simulink model "gm_FCS_MPC_3Phase_SPMSM_TEST1"  (R2022a)
settings: Solver=ode23t  StartTime=0.0  StopTime=0.2  RelTol=1e-3  AbsTol=1e-3  EnableMultiTasking=on
undefined symbols (not defined in the file or in its folder): f_c, Ld, Lq, np, psiPM, R, T_50MHz, u_dc
libraries: hdlmdlgenlib x26, ee_lib x22, nesl_utility x22, fl_lib x21, simulink x7
(part 4 of 5)

== system gm_FCS_MPC_3Phase_SPMSM_TEST1/Microcontroller Software/Subsystem1/MATLAB Function/adder25 ==
  In1 : Inport
  In2 : Inport  Port=2
  adder25 : Sum  OutDataTypeStr=single  SampleTime=1e-08
  Out1 : Outport
  wires:
  In1/1 -> adder25/1
  In2/1 -> adder25/2
  adder25/1 -> Out1/1

== system gm_FCS_MPC_3Phase_SPMSM_TEST1/Microcontroller Software/Subsystem1/MATLAB Function/adder26 ==
  In1 : Inport
  In2 : Inport  Port=2
  adder26 : Sum  OutDataTypeStr=single  SampleTime=1e-08
  Out1 : Outport
  wires:
  In1/1 -> adder26/1
  In2/1 -> adder26/2
  adder26/1 -> Out1/1

== system gm_FCS_MPC_3Phase_SPMSM_TEST1/Microcontroller Software/Subsystem1/MATLAB Function/adder27 ==
  In1 : Inport
  In2 : Inport  Port=2
  adder27 : Sum  OutDataTypeStr=single  SampleTime=1e-08
  Out1 : Outport
  wires:
  In1/1 -> adder27/1
  In2/1 -> adder27/2
  adder27/1 -> Out1/1

== system gm_FCS_MPC_3Phase_SPMSM_TEST1/Microcontroller Software/Subsystem1/MATLAB Function/adder28 ==
  In1 : Inport
  In2 : Inport  Port=2
  adder28 : Sum  OutDataTypeStr=single  SampleTime=1e-08
  Out1 : Outport
  wires:
  In1/1 -> adder28/1
  In2/1 -> adder28/2
  adder28/1 -> Out1/1

== system gm_FCS_MPC_3Phase_SPMSM_TEST1/Microcontroller Software/Subsystem1/MATLAB Function/adder29 ==
  In1 : Inport
  In2 : Inport  Port=2
  adder29 : Sum  OutDataTypeStr=single  SampleTime=1e-08
  Out1 : Outport
  wires:
  In1/1 -> adder29/1
  In2/1 -> adder29/2
  adder29/1 -> Out1/1

== system gm_FCS_MPC_3Phase_SPMSM_TEST1/Microcontroller Software/Subsystem1/MATLAB Function/adder3 ==
  In1 : Inport
  In2 : Inport  Port=2
  adder3 : Sum  OutDataTypeStr=single  SampleTime=1e-08
  Out1 : Outport
  wires:
  In1/1 -> adder3/1
  In2/1 -> adder3/2
  adder3/1 -> Out1/1

== system gm_FCS_MPC_3Phase_SPMSM_TEST1/Microcontroller Software/Subsystem1/MATLAB Function/adder30 ==
  In1 : Inport
  In2 : Inport  Port=2
  adder30 : Sum  OutDataTypeStr=single  SampleTime=1e-08
  Out1 : Outport
  wires:
  In1/1 -> adder30/1
  In2/1 -> adder30/2
  adder30/1 -> Out1/1

== system gm_FCS_MPC_3Phase_SPMSM_TEST1/Microcontroller Software/Subsystem1/MATLAB Function/adder31 ==
  In1 : Inport
  In2 : Inport  Port=2
  adder31 : Sum  OutDataTypeStr=single  SampleTime=1e-08
  Out1 : Outport
  wires:
  In1/1 -> adder31/1
  In2/1 -> adder31/2
  adder31/1 -> Out1/1

== system gm_FCS_MPC_3Phase_SPMSM_TEST1/Microcontroller Software/Subsystem1/MATLAB Function/adder32 ==
  In1 : Inport
  In2 : Inport  Port=2
  adder32 : Sum  OutDataTypeStr=single  SampleTime=1e-08
  Out1 : Outport
  wires:
  In1/1 -> adder32/1
  In2/1 -> adder32/2
  adder32/1 -> Out1/1

== system gm_FCS_MPC_3Phase_SPMSM_TEST1/Microcontroller Software/Subsystem1/MATLAB Function/adder33 ==
  In1 : Inport
  In2 : Inport  Port=2
  adder33 : Sum  OutDataTypeStr=single  SampleTime=1e-08
  Out1 : Outport
  wires:
  In1/1 -> adder33/1
  In2/1 -> adder33/2
  adder33/1 -> Out1/1

== system gm_FCS_MPC_3Phase_SPMSM_TEST1/Microcontroller Software/Subsystem1/MATLAB Function/adder34 ==
  In1 : Inport
  In2 : Inport  Port=2
  adder34 : Sum  OutDataTypeStr=single  SampleTime=1e-08
  Out1 : Outport
  wires:
  In1/1 -> adder34/1
  In2/1 -> adder34/2
  adder34/1 -> Out1/1

== system gm_FCS_MPC_3Phase_SPMSM_TEST1/Microcontroller Software/Subsystem1/MATLAB Function/adder4 ==
  In1 : Inport
  In2 : Inport  Port=2
  adder4 : Sum  OutDataTypeStr=single  SampleTime=1e-08
  Out1 : Outport
  wires:
  In1/1 -> adder4/1
  In2/1 -> adder4/2
  adder4/1 -> Out1/1

== system gm_FCS_MPC_3Phase_SPMSM_TEST1/Microcontroller Software/Subsystem1/MATLAB Function/adder5 ==
  In1 : Inport
  In2 : Inport  Port=2
  adder5 : Sum  OutDataTypeStr=single  SampleTime=1e-08
  Out1 : Outport
  wires:
  In1/1 -> adder5/1
  In2/1 -> adder5/2
  adder5/1 -> Out1/1

== system gm_FCS_MPC_3Phase_SPMSM_TEST1/Microcontroller Software/Subsystem1/MATLAB Function/adder6 ==
  In1 : Inport
  In2 : Inport  Port=2
  adder6 : Sum  OutDataTypeStr=single  SampleTime=1e-08
  Out1 : Outport
  wires:
  In1/1 -> adder6/1
  In2/1 -> adder6/2
  adder6/1 -> Out1/1

== system gm_FCS_MPC_3Phase_SPMSM_TEST1/Microcontroller Software/Subsystem1/MATLAB Function/adder7 ==
  In1 : Inport
  In2 : Inport  Port=2
  adder7 : Sum  OutDataTypeStr=single  SampleTime=1e-08
  Out1 : Outport
  wires:
  In1/1 -> adder7/1
  In2/1 -> adder7/2
  adder7/1 -> Out1/1

== system gm_FCS_MPC_3Phase_SPMSM_TEST1/Microcontroller Software/Subsystem1/MATLAB Function/adder8 ==
  In1 : Inport
  In2 : Inport  Port=2
  adder8 : Sum  OutDataTypeStr=single  SampleTime=1e-08
  Out1 : Outport
  wires:
  In1/1 -> adder8/1
  In2/1 -> adder8/2
  adder8/1 -> Out1/1

== system gm_FCS_MPC_3Phase_SPMSM_TEST1/Microcontroller Software/Subsystem1/MATLAB Function/adder9 ==
  In1 : Inport
  In2 : Inport  Port=2
  adder9 : Sum  OutDataTypeStr=single  SampleTime=1e-08
  Out1 : Outport
  wires:
  In1/1 -> adder9/1
  In2/1 -> adder9/2
  adder9/1 -> Out1/1

== system gm_FCS_MPC_3Phase_SPMSM_TEST1/Microcontroller Software/Subsystem1/MATLAB Function/cos_to_sincos ==
  In1 : Inport
  cos_to_sincos : Trigonometry  Operator=sincos  SampleTime=1e-08
  Out1 : Outport
  Out2 : Outport  Port=2
  wires:
  In1/1 -> cos_to_sincos/1
  cos_to_sincos/1 -> Out1/1
  cos_to_sincos/2 -> Out2/1

== system gm_FCS_MPC_3Phase_SPMSM_TEST1/Microcontroller Software/Subsystem1/MATLAB Function/divider ==
  In1 : Inport
  In2 : Inport  Port=2
  divider : Product  Inputs=*/  OutDataTypeStr=single  SampleTime=1e-08
  Out1 : Outport
  wires:
  In1/1 -> divider/1
  In2/1 -> divider/2
  divider/1 -> Out1/1

== system gm_FCS_MPC_3Phase_SPMSM_TEST1/Microcontroller Software/Subsystem1/MATLAB Function/divider1 ==
  In1 : Inport
  In2 : Inport  Port=2
  divider1 : Product  Inputs=*/  OutDataTypeStr=single  SampleTime=1e-08
  Out1 : Outport
  wires:
  In1/1 -> divider1/1
  In2/1 -> divider1/2
  divider1/1 -> Out1/1

== system gm_FCS_MPC_3Phase_SPMSM_TEST1/Microcontroller Software/Subsystem1/MATLAB Function/divider10 ==
  In1 : Inport
  In2 : Inport  Port=2
  divider10 : Product  Inputs=*/  OutDataTypeStr=single  SampleTime=1e-08
  Out1 : Outport
  wires:
  In1/1 -> divider10/1
  In2/1 -> divider10/2
  divider10/1 -> Out1/1

== system gm_FCS_MPC_3Phase_SPMSM_TEST1/Microcontroller Software/Subsystem1/MATLAB Function/divider11 ==
  In1 : Inport
  In2 : Inport  Port=2
  divider11 : Product  Inputs=*/  OutDataTypeStr=single  SampleTime=1e-08
  Out1 : Outport
  wires:
  In1/1 -> divider11/1
  In2/1 -> divider11/2
  divider11/1 -> Out1/1

== system gm_FCS_MPC_3Phase_SPMSM_TEST1/Microcontroller Software/Subsystem1/MATLAB Function/divider12 ==
  In1 : Inport
  In2 : Inport  Port=2
  divider12 : Product  Inputs=*/  OutDataTypeStr=single  SampleTime=1e-08
  Out1 : Outport
  wires:
  In1/1 -> divider12/1
  In2/1 -> divider12/2
  divider12/1 -> Out1/1

== system gm_FCS_MPC_3Phase_SPMSM_TEST1/Microcontroller Software/Subsystem1/MATLAB Function/divider13 ==
  In1 : Inport
  In2 : Inport  Port=2
  divider13 : Product  Inputs=*/  OutDataTypeStr=single  SampleTime=1e-08
  Out1 : Outport
  wires:
  In1/1 -> divider13/1
  In2/1 -> divider13/2
  divider13/1 -> Out1/1

== system gm_FCS_MPC_3Phase_SPMSM_TEST1/Microcontroller Software/Subsystem1/MATLAB Function/divider14 ==
  In1 : Inport
  In2 : Inport  Port=2
  divider14 : Product  Inputs=*/  OutDataTypeStr=single  SampleTime=1e-08
  Out1 : Outport
  wires:
  In1/1 -> divider14/1
  In2/1 -> divider14/2
  divider14/1 -> Out1/1

== system gm_FCS_MPC_3Phase_SPMSM_TEST1/Microcontroller Software/Subsystem1/MATLAB Function/divider15 ==
  In1 : Inport
  In2 : Inport  Port=2
  divider15 : Product  Inputs=*/  OutDataTypeStr=single  SampleTime=1e-08
  Out1 : Outport
  wires:
  In1/1 -> divider15/1
  In2/1 -> divider15/2
  divider15/1 -> Out1/1

== system gm_FCS_MPC_3Phase_SPMSM_TEST1/Microcontroller Software/Subsystem1/MATLAB Function/divider16 ==
  In1 : Inport
  In2 : Inport  Port=2
  divider16 : Product  Inputs=*/  OutDataTypeStr=single  SampleTime=1e-08
  Out1 : Outport
  wires:
  In1/1 -> divider16/1
  In2/1 -> divider16/2
  divider16/1 -> Out1/1

== system gm_FCS_MPC_3Phase_SPMSM_TEST1/Microcontroller Software/Subsystem1/MATLAB Function/divider17 ==
  In1 : Inport
  In2 : Inport  Port=2
  divider17 : Product  Inputs=*/  OutDataTypeStr=single  SampleTime=1e-08
  Out1 : Outport
  wires:
  In1/1 -> divider17/1
  In2/1 -> divider17/2
  divider17/1 -> Out1/1

== system gm_FCS_MPC_3Phase_SPMSM_TEST1/Microcontroller Software/Subsystem1/MATLAB Function/divider18 ==
  In1 : Inport
  In2 : Inport  Port=2
  divider18 : Product  Inputs=*/  OutDataTypeStr=single  SampleTime=1e-08
  Out1 : Outport
  wires:
  In1/1 -> divider18/1
  In2/1 -> divider18/2
  divider18/1 -> Out1/1

== system gm_FCS_MPC_3Phase_SPMSM_TEST1/Microcontroller Software/Subsystem1/MATLAB Function/divider19 ==
  In1 : Inport
  In2 : Inport  Port=2
  divider19 : Product  Inputs=*/  OutDataTypeStr=single  SampleTime=1e-08
  Out1 : Outport
  wires:
  In1/1 -> divider19/1
  In2/1 -> divider19/2
  divider19/1 -> Out1/1

== system gm_FCS_MPC_3Phase_SPMSM_TEST1/Microcontroller Software/Subsystem1/MATLAB Function/divider2 ==
  In1 : Inport
  In2 : Inport  Port=2
  divider2 : Product  Inputs=*/  OutDataTypeStr=single  SampleTime=1e-08
  Out1 : Outport
  wires:
  In1/1 -> divider2/1
  In2/1 -> divider2/2
  divider2/1 -> Out1/1

== system gm_FCS_MPC_3Phase_SPMSM_TEST1/Microcontroller Software/Subsystem1/MATLAB Function/divider20 ==
  In1 : Inport
  In2 : Inport  Port=2
  divider20 : Product  Inputs=*/  OutDataTypeStr=single  SampleTime=1e-08
  Out1 : Outport
  wires:
  In1/1 -> divider20/1
  In2/1 -> divider20/2
  divider20/1 -> Out1/1

== system gm_FCS_MPC_3Phase_SPMSM_TEST1/Microcontroller Software/Subsystem1/MATLAB Function/divider21 ==
  In1 : Inport
  In2 : Inport  Port=2
  divider21 : Product  Inputs=*/  OutDataTypeStr=single  SampleTime=1e-08
  Out1 : Outport
  wires:
  In1/1 -> divider21/1
  In2/1 -> divider21/2
  divider21/1 -> Out1/1

== system gm_FCS_MPC_3Phase_SPMSM_TEST1/Microcontroller Software/Subsystem1/MATLAB Function/divider22 ==
  In1 : Inport
  In2 : Inport  Port=2
  divider22 : Product  Inputs=*/  OutDataTypeStr=single  SampleTime=1e-08
  Out1 : Outport
  wires:
  In1/1 -> divider22/1
  In2/1 -> divider22/2
  divider22/1 -> Out1/1

== system gm_FCS_MPC_3Phase_SPMSM_TEST1/Microcontroller Software/Subsystem1/MATLAB Function/divider23 ==
  In1 : Inport
  In2 : Inport  Port=2
  divider23 : Product  Inputs=*/  OutDataTypeStr=single  SampleTime=1e-08
  Out1 : Outport
  wires:
  In1/1 -> divider23/1
  In2/1 -> divider23/2
  divider23/1 -> Out1/1

== system gm_FCS_MPC_3Phase_SPMSM_TEST1/Microcontroller Software/Subsystem1/MATLAB Function/divider24 ==
  In1 : Inport
  In2 : Inport  Port=2
  divider24 : Product  Inputs=*/  OutDataTypeStr=single  SampleTime=1e-08
  Out1 : Outport
  wires:
  In1/1 -> divider24/1
  In2/1 -> divider24/2
  divider24/1 -> Out1/1

== system gm_FCS_MPC_3Phase_SPMSM_TEST1/Microcontroller Software/Subsystem1/MATLAB Function/divider25 ==
  In1 : Inport
  In2 : Inport  Port=2
  divider25 : Product  Inputs=*/  OutDataTypeStr=single  SampleTime=1e-08
  Out1 : Outport
  wires:
  In1/1 -> divider25/1
  In2/1 -> divider25/2
  divider25/1 -> Out1/1

== system gm_FCS_MPC_3Phase_SPMSM_TEST1/Microcontroller Software/Subsystem1/MATLAB Function/divider26 ==
  In1 : Inport
  In2 : Inport  Port=2
  divider26 : Product  Inputs=*/  OutDataTypeStr=single  SampleTime=1e-08
  Out1 : Outport
  wires:
  In1/1 -> divider26/1
  In2/1 -> divider26/2
  divider26/1 -> Out1/1

== system gm_FCS_MPC_3Phase_SPMSM_TEST1/Microcontroller Software/Subsystem1/MATLAB Function/divider27 ==
  In1 : Inport
  In2 : Inport  Port=2
  divider27 : Product  Inputs=*/  OutDataTypeStr=single  SampleTime=1e-08
  Out1 : Outport
  wires:
  In1/1 -> divider27/1
  In2/1 -> divider27/2
  divider27/1 -> Out1/1

== system gm_FCS_MPC_3Phase_SPMSM_TEST1/Microcontroller Software/Subsystem1/MATLAB Function/divider28 ==
  In1 : Inport
  In2 : Inport  Port=2
  divider28 : Product  Inputs=*/  OutDataTypeStr=single  SampleTime=1e-08
  Out1 : Outport
  wires:
  In1/1 -> divider28/1
  In2/1 -> divider28/2
  divider28/1 -> Out1/1

== system gm_FCS_MPC_3Phase_SPMSM_TEST1/Microcontroller Software/Subsystem1/MATLAB Function/divider29 ==
  In1 : Inport
  In2 : Inport  Port=2
  divider29 : Product  Inputs=*/  OutDataTypeStr=single  SampleTime=1e-08
  Out1 : Outport
  wires:
  In1/1 -> divider29/1
  In2/1 -> divider29/2
  divider29/1 -> Out1/1

== system gm_FCS_MPC_3Phase_SPMSM_TEST1/Microcontroller Software/Subsystem1/MATLAB Function/divider3 ==
  In1 : Inport
  In2 : Inport  Port=2
  divider3 : Product  Inputs=*/  OutDataTypeStr=single  SampleTime=1e-08
  Out1 : Outport
  wires:
  In1/1 -> divider3/1
  In2/1 -> divider3/2
  divider3/1 -> Out1/1

== system gm_FCS_MPC_3Phase_SPMSM_TEST1/Microcontroller Software/Subsystem1/MATLAB Function/divider30 ==
  In1 : Inport
  In2 : Inport  Port=2
  divider30 : Product  Inputs=*/  OutDataTypeStr=single  SampleTime=1e-08
  Out1 : Outport
  wires:
  In1/1 -> divider30/1
  In2/1 -> divider30/2
  divider30/1 -> Out1/1

== system gm_FCS_MPC_3Phase_SPMSM_TEST1/Microcontroller Software/Subsystem1/MATLAB Function/divider31 ==
  In1 : Inport
  In2 : Inport  Port=2
  divider31 : Product  Inputs=*/  OutDataTypeStr=single  SampleTime=1e-08
  Out1 : Outport
  wires:
  In1/1 -> divider31/1
  In2/1 -> divider31/2
  divider31/1 -> Out1/1

== system gm_FCS_MPC_3Phase_SPMSM_TEST1/Microcontroller Software/Subsystem1/MATLAB Function/divider32 ==
  In1 : Inport
  In2 : Inport  Port=2
  divider32 : Product  Inputs=*/  OutDataTypeStr=single  SampleTime=1e-08
  Out1 : Outport
  wires:
  In1/1 -> divider32/1
  In2/1 -> divider32/2
  divider32/1 -> Out1/1

== system gm_FCS_MPC_3Phase_SPMSM_TEST1/Microcontroller Software/Subsystem1/MATLAB Function/divider33 ==
  In1 : Inport
  In2 : Inport  Port=2
  divider33 : Product  Inputs=*/  OutDataTypeStr=single  SampleTime=1e-08
  Out1 : Outport
  wires:
  In1/1 -> divider33/1
  In2/1 -> divider33/2
  divider33/1 -> Out1/1

== system gm_FCS_MPC_3Phase_SPMSM_TEST1/Microcontroller Software/Subsystem1/MATLAB Function/divider34 ==
  In1 : Inport
  In2 : Inport  Port=2
  divider34 : Product  Inputs=*/  OutDataTypeStr=single  SampleTime=1e-08
  Out1 : Outport
  wires:
  In1/1 -> divider34/1
  In2/1 -> divider34/2
  divider34/1 -> Out1/1

== system gm_FCS_MPC_3Phase_SPMSM_TEST1/Microcontroller Software/Subsystem1/MATLAB Function/divider35 ==
  In1 : Inport
  In2 : Inport  Port=2
  divider35 : Product  Inputs=*/  OutDataTypeStr=single  SampleTime=1e-08
  Out1 : Outport
  wires:
  In1/1 -> divider35/1
  In2/1 -> divider35/2
  divider35/1 -> Out1/1

== system gm_FCS_MPC_3Phase_SPMSM_TEST1/Microcontroller Software/Subsystem1/MATLAB Function/divider4 ==
  In1 : Inport
  In2 : Inport  Port=2
  divider4 : Product  Inputs=*/  OutDataTypeStr=single  SampleTime=1e-08
  Out1 : Outport
  wires:
  In1/1 -> divider4/1
  In2/1 -> divider4/2
  divider4/1 -> Out1/1

== system gm_FCS_MPC_3Phase_SPMSM_TEST1/Microcontroller Software/Subsystem1/MATLAB Function/divider5 ==
  In1 : Inport
  In2 : Inport  Port=2
  divider5 : Product  Inputs=*/  OutDataTypeStr=single  SampleTime=1e-08
  Out1 : Outport
  wires:
  In1/1 -> divider5/1
  In2/1 -> divider5/2
  divider5/1 -> Out1/1

== system gm_FCS_MPC_3Phase_SPMSM_TEST1/Microcontroller Software/Subsystem1/MATLAB Function/divider6 ==
  In1 : Inport
  In2 : Inport  Port=2
  divider6 : Product  Inputs=*/  OutDataTypeStr=single  SampleTime=1e-08
  Out1 : Outport
  wires:
  In1/1 -> divider6/1
  In2/1 -> divider6/2
  divider6/1 -> Out1/1

== system gm_FCS_MPC_3Phase_SPMSM_TEST1/Microcontroller Software/Subsystem1/MATLAB Function/divider7 ==
  In1 : Inport
  In2 : Inport  Port=2
  divider7 : Product  Inputs=*/  OutDataTypeStr=single  SampleTime=1e-08
  Out1 : Outport
  wires:
  In1/1 -> divider7/1
  In2/1 -> divider7/2
  divider7/1 -> Out1/1

== system gm_FCS_MPC_3Phase_SPMSM_TEST1/Microcontroller Software/Subsystem1/MATLAB Function/divider8 ==
  In1 : Inport
  In2 : Inport  Port=2
  divider8 : Product  Inputs=*/  OutDataTypeStr=single  SampleTime=1e-08
  Out1 : Outport
  wires:
  In1/1 -> divider8/1
  In2/1 -> divider8/2
  divider8/1 -> Out1/1

== system gm_FCS_MPC_3Phase_SPMSM_TEST1/Microcontroller Software/Subsystem1/MATLAB Function/divider9 ==
  In1 : Inport
  In2 : Inport  Port=2
  divider9 : Product  Inputs=*/  OutDataTypeStr=single  SampleTime=1e-08
  Out1 : Outport
  wires:
  In1/1 -> divider9/1
  In2/1 -> divider9/2
  divider9/1 -> Out1/1

== system gm_FCS_MPC_3Phase_SPMSM_TEST1/Microcontroller Software/Subsystem1/MATLAB Function/dtc ==
  In1 : Inport
  dtc : DataTypeConversion  OutDataTypeStr=double  SampleTime=1e-08  SaturateOnIntegerOverflow=off  RndMeth=Floor
  Out1 : Outport
  wires:
  In1/1 -> dtc/1
  dtc/1 -> Out1/1

== system gm_FCS_MPC_3Phase_SPMSM_TEST1/Microcontroller Software/Subsystem1/MATLAB Function/dtc1 ==
  In1 : Inport
  dtc1 : DataTypeConversion  OutDataTypeStr=double  SampleTime=1e-08  SaturateOnIntegerOverflow=off  RndMeth=Floor
  Out1 : Outport
  wires:
  In1/1 -> dtc1/1
  dtc1/1 -> Out1/1

== system gm_FCS_MPC_3Phase_SPMSM_TEST1/Microcontroller Software/Subsystem1/MATLAB Function/dtc2 ==
  In1 : Inport
  dtc2 : DataTypeConversion  OutDataTypeStr=double  SampleTime=1e-08  SaturateOnIntegerOverflow=off  RndMeth=Floor
  Out1 : Outport
  wires:
  In1/1 -> dtc2/1
  dtc2/1 -> Out1/1

== system gm_FCS_MPC_3Phase_SPMSM_TEST1/Microcontroller Software/Subsystem1/MATLAB Function/dtc3 ==
  In1 : Inport
  dtc3 : DataTypeConversion  OutDataTypeStr=double  SampleTime=1e-08  SaturateOnIntegerOverflow=off  RndMeth=Floor
  Out1 : Outport
  wires:
  In1/1 -> dtc3/1
  dtc3/1 -> Out1/1

== system gm_FCS_MPC_3Phase_SPMSM_TEST1/Microcontroller Software/Subsystem1/MATLAB Function/dtc4 ==
  In1 : Inport
  dtc4 : DataTypeConversion  OutDataTypeStr=double  SampleTime=1e-08  SaturateOnIntegerOverflow=off  RndMeth=Floor
  Out1 : Outport
  wires:
  In1/1 -> dtc4/1
  dtc4/1 -> Out1/1

== system gm_FCS_MPC_3Phase_SPMSM_TEST1/Microcontroller Software/Subsystem1/MATLAB Function/dtc5 ==
  In1 : Inport
  dtc5 : DataTypeConversion  OutDataTypeStr=double  SampleTime=1e-08  SaturateOnIntegerOverflow=off  RndMeth=Floor
  Out1 : Outport
  wires:
  In1/1 -> dtc5/1
  dtc5/1 -> Out1/1

== system gm_FCS_MPC_3Phase_SPMSM_TEST1/Microcontroller Software/Subsystem1/MATLAB Function/dtc6 ==
  In1 : Inport
  dtc6 : DataTypeConversion  OutDataTypeStr=double  SampleTime=1e-08  SaturateOnIntegerOverflow=off  RndMeth=Floor
  Out1 : Outport
  wires:
  In1/1 -> dtc6/1
  dtc6/1 -> Out1/1

== system gm_FCS_MPC_3Phase_SPMSM_TEST1/Microcontroller Software/Subsystem1/MATLAB Function/dtc7 ==
  In1 : Inport
  dtc7 : DataTypeConversion  OutDataTypeStr=double  SampleTime=1e-08  SaturateOnIntegerOverflow=off  RndMeth=Floor
  Out1 : Outport
  wires:
  In1/1 -> dtc7/1
  dtc7/1 -> Out1/1

== system gm_FCS_MPC_3Phase_SPMSM_TEST1/Microcontroller Software/Subsystem1/MATLAB Function/gain1 ==
  In1 : Inport
  In2 : Inport  Port=2
  gain1 : Product  Inputs=**  OutDataTypeStr=single  SampleTime=1e-08
  Out1 : Outport
  wires:
  In1/1 -> gain1/1
  In2/1 -> gain1/2
  gain1/1 -> Out1/1

== system gm_FCS_MPC_3Phase_SPMSM_TEST1/Microcontroller Software/Subsystem1/MATLAB Function/multiplier ==
  In1 : Inport
  In2 : Inport  Port=2
  multiplier : Product  Inputs=**  OutDataTypeStr=single  SampleTime=1e-08
  Out1 : Outport
  wires:
  In1/1 -> multiplier/1
  In2/1 -> multiplier/2
  multiplier/1 -> Out1/1

== system gm_FCS_MPC_3Phase_SPMSM_TEST1/Microcontroller Software/Subsystem1/MATLAB Function/multiplier1 ==
  In1 : Inport
  In2 : Inport  Port=2
  multiplier1 : Product  Inputs=**  OutDataTypeStr=single  SampleTime=1e-08
  Out1 : Outport
  wires:
  In1/1 -> multiplier1/1
  In2/1 -> multiplier1/2
  multiplier1/1 -> Out1/1

== system gm_FCS_MPC_3Phase_SPMSM_TEST1/Microcontroller Software/Subsystem1/MATLAB Function/multiplier10 ==
  In1 : Inport
  In2 : Inport  Port=2
  multiplier10 : Product  Inputs=**  OutDataTypeStr=single  SampleTime=1e-08
  Out1 : Outport
  wires:
  In1/1 -> multiplier10/1
  In2/1 -> multiplier10/2
  multiplier10/1 -> Out1/1

== system gm_FCS_MPC_3Phase_SPMSM_TEST1/Microcontroller Software/Subsystem1/MATLAB Function/multiplier11 ==
  In1 : Inport
  In2 : Inport  Port=2
  multiplier11 : Product  Inputs=**  OutDataTypeStr=single  SampleTime=1e-08
  Out1 : Outport
  wires:
  In1/1 -> multiplier11/1
  In2/1 -> multiplier11/2
  multiplier11/1 -> Out1/1

== system gm_FCS_MPC_3Phase_SPMSM_TEST1/Microcontroller Software/Subsystem1/MATLAB Function/multiplier12 ==
  In1 : Inport
  In2 : Inport  Port=2
  multiplier12 : Product  Inputs=**  OutDataTypeStr=single  SampleTime=1e-08
  Out1 : Outport
  wires:
  In1/1 -> multiplier12/1
  In2/1 -> multiplier12/2
  multiplier12/1 -> Out1/1

== system gm_FCS_MPC_3Phase_SPMSM_TEST1/Microcontroller Software/Subsystem1/MATLAB Function/multiplier13 ==
  In1 : Inport
  In2 : Inport  Port=2
  multiplier13 : Product  Inputs=**  OutDataTypeStr=single  SampleTime=1e-08
  Out1 : Outport
  wires:
  In1/1 -> multiplier13/1
  In2/1 -> multiplier13/2
  multiplier13/1 -> Out1/1

== system gm_FCS_MPC_3Phase_SPMSM_TEST1/Microcontroller Software/Subsystem1/MATLAB Function/multiplier14 ==
  In1 : Inport
  In2 : Inport  Port=2
  multiplier14 : Product  Inputs=**  OutDataTypeStr=single  SampleTime=1e-08
  Out1 : Outport
  wires:
  In1/1 -> multiplier14/1
  In2/1 -> multiplier14/2
  multiplier14/1 -> Out1/1

== system gm_FCS_MPC_3Phase_SPMSM_TEST1/Microcontroller Software/Subsystem1/MATLAB Function/multiplier15 ==
  In1 : Inport
  In2 : Inport  Port=2
  multiplier15 : Product  Inputs=**  OutDataTypeStr=single  SampleTime=1e-08
  Out1 : Outport
  wires:
  In1/1 -> multiplier15/1
  In2/1 -> multiplier15/2
  multiplier15/1 -> Out1/1

== system gm_FCS_MPC_3Phase_SPMSM_TEST1/Microcontroller Software/Subsystem1/MATLAB Function/multiplier16 ==
  In1 : Inport
  In2 : Inport  Port=2
  multiplier16 : Product  Inputs=**  OutDataTypeStr=single  SampleTime=1e-08
  Out1 : Outport
  wires:
  In1/1 -> multiplier16/1
  In2/1 -> multiplier16/2
  multiplier16/1 -> Out1/1

== system gm_FCS_MPC_3Phase_SPMSM_TEST1/Microcontroller Software/Subsystem1/MATLAB Function/multiplier17 ==
  In1 : Inport
  In2 : Inport  Port=2
  multiplier17 : Product  Inputs=**  OutDataTypeStr=single  SampleTime=1e-08
  Out1 : Outport
  wires:
  In1/1 -> multiplier17/1
  In2/1 -> multiplier17/2
  multiplier17/1 -> Out1/1

== system gm_FCS_MPC_3Phase_SPMSM_TEST1/Microcontroller Software/Subsystem1/MATLAB Function/multiplier18 ==
  In1 : Inport
  In2 : Inport  Port=2
  multiplier18 : Product  Inputs=**  OutDataTypeStr=single  SampleTime=1e-08
  Out1 : Outport
  wires:
  In1/1 -> multiplier18/1
  In2/1 -> multiplier18/2
  multiplier18/1 -> Out1/1

== system gm_FCS_MPC_3Phase_SPMSM_TEST1/Microcontroller Software/Subsystem1/MATLAB Function/multiplier19 ==
  In1 : Inport
  In2 : Inport  Port=2
  multiplier19 : Product  Inputs=**  OutDataTypeStr=single  SampleTime=1e-08
  Out1 : Outport
  wires:
  In1/1 -> multiplier19/1
  In2/1 -> multiplier19/2
  multiplier19/1 -> Out1/1

== system gm_FCS_MPC_3Phase_SPMSM_TEST1/Microcontroller Software/Subsystem1/MATLAB Function/multiplier2 ==
  In1 : Inport
  In2 : Inport  Port=2
  multiplier2 : Product  Inputs=**  OutDataTypeStr=single  SampleTime=1e-08
  Out1 : Outport
  wires:
  In1/1 -> multiplier2/1
  In2/1 -> multiplier2/2
  multiplier2/1 -> Out1/1

== system gm_FCS_MPC_3Phase_SPMSM_TEST1/Microcontroller Software/Subsystem1/MATLAB Function/multiplier20 ==
  In1 : Inport
  In2 : Inport  Port=2
  multiplier20 : Product  Inputs=**  OutDataTypeStr=single  SampleTime=1e-08
  Out1 : Outport
  wires:
  In1/1 -> multiplier20/1
  In2/1 -> multiplier20/2
  multiplier20/1 -> Out1/1

== system gm_FCS_MPC_3Phase_SPMSM_TEST1/Microcontroller Software/Subsystem1/MATLAB Function/multiplier21 ==
  In1 : Inport
  In2 : Inport  Port=2
  multiplier21 : Product  Inputs=**  OutDataTypeStr=single  SampleTime=1e-08
  Out1 : Outport
  wires:
  In1/1 -> multiplier21/1
  In2/1 -> multiplier21/2
  multiplier21/1 -> Out1/1

== system gm_FCS_MPC_3Phase_SPMSM_TEST1/Microcontroller Software/Subsystem1/MATLAB Function/multiplier22 ==
  In1 : Inport
  In2 : Inport  Port=2
  multiplier22 : Product  Inputs=**  OutDataTypeStr=single  SampleTime=1e-08
  Out1 : Outport
  wires:
  In1/1 -> multiplier22/1
  In2/1 -> multiplier22/2
  multiplier22/1 -> Out1/1

== system gm_FCS_MPC_3Phase_SPMSM_TEST1/Microcontroller Software/Subsystem1/MATLAB Function/multiplier23 ==
  In1 : Inport
  In2 : Inport  Port=2
  multiplier23 : Product  Inputs=**  OutDataTypeStr=single  SampleTime=1e-08
  Out1 : Outport
  wires:
  In1/1 -> multiplier23/1
  In2/1 -> multiplier23/2
  multiplier23/1 -> Out1/1

== system gm_FCS_MPC_3Phase_SPMSM_TEST1/Microcontroller Software/Subsystem1/MATLAB Function/multiplier24 ==
  In1 : Inport
  In2 : Inport  Port=2
  multiplier24 : Product  Inputs=**  OutDataTypeStr=single  SampleTime=1e-08
  Out1 : Outport
  wires:
  In1/1 -> multiplier24/1
  In2/1 -> multiplier24/2
  multiplier24/1 -> Out1/1

== system gm_FCS_MPC_3Phase_SPMSM_TEST1/Microcontroller Software/Subsystem1/MATLAB Function/multiplier25 ==
  In1 : Inport
  In2 : Inport  Port=2
  multiplier25 : Product  Inputs=**  OutDataTypeStr=single  SampleTime=1e-08
  Out1 : Outport
  wires:
  In1/1 -> multiplier25/1
  In2/1 -> multiplier25/2
  multiplier25/1 -> Out1/1

== system gm_FCS_MPC_3Phase_SPMSM_TEST1/Microcontroller Software/Subsystem1/MATLAB Function/multiplier26 ==
  In1 : Inport
  In2 : Inport  Port=2
  multiplier26 : Product  Inputs=**  OutDataTypeStr=single  SampleTime=1e-08
  Out1 : Outport
  wires:
  In1/1 -> multiplier26/1
  In2/1 -> multiplier26/2
  multiplier26/1 -> Out1/1

== system gm_FCS_MPC_3Phase_SPMSM_TEST1/Microcontroller Software/Subsystem1/MATLAB Function/multiplier27 ==
  In1 : Inport
  In2 : Inport  Port=2
  multiplier27 : Product  Inputs=**  OutDataTypeStr=single  SampleTime=1e-08
  Out1 : Outport
  wires:
  In1/1 -> multiplier27/1
  In2/1 -> multiplier27/2
  multiplier27/1 -> Out1/1

== system gm_FCS_MPC_3Phase_SPMSM_TEST1/Microcontroller Software/Subsystem1/MATLAB Function/multiplier28 ==
  In1 : Inport
  In2 : Inport  Port=2
  multiplier28 : Product  Inputs=**  OutDataTypeStr=single  SampleTime=1e-08
  Out1 : Outport
  wires:
  In1/1 -> multiplier28/1
  In2/1 -> multiplier28/2
  multiplier28/1 -> Out1/1

== system gm_FCS_MPC_3Phase_SPMSM_TEST1/Microcontroller Software/Subsystem1/MATLAB Function/multiplier29 ==
  In1 : Inport
  In2 : Inport  Port=2
  multiplier29 : Product  Inputs=**  OutDataTypeStr=single  SampleTime=1e-08
  Out1 : Outport
  wires:
  In1/1 -> multiplier29/1
  In2/1 -> multiplier29/2
  multiplier29/1 -> Out1/1

== system gm_FCS_MPC_3Phase_SPMSM_TEST1/Microcontroller Software/Subsystem1/MATLAB Function/multiplier3 ==
  In1 : Inport
  In2 : Inport  Port=2
  multiplier3 : Product  Inputs=**  OutDataTypeStr=single  SampleTime=1e-08
  Out1 : Outport
  wires:
  In1/1 -> multiplier3/1
  In2/1 -> multiplier3/2
  multiplier3/1 -> Out1/1

== system gm_FCS_MPC_3Phase_SPMSM_TEST1/Microcontroller Software/Subsystem1/MATLAB Function/multiplier30 ==
  In1 : Inport
  In2 : Inport  Port=2
  multiplier30 : Product  Inputs=**  OutDataTypeStr=single  SampleTime=1e-08
  Out1 : Outport
  wires:
  In1/1 -> multiplier30/1
  In2/1 -> multiplier30/2
  multiplier30/1 -> Out1/1

== system gm_FCS_MPC_3Phase_SPMSM_TEST1/Microcontroller Software/Subsystem1/MATLAB Function/multiplier31 ==
  In1 : Inport
  In2 : Inport  Port=2
  multiplier31 : Product  Inputs=**  OutDataTypeStr=single  SampleTime=1e-08
  Out1 : Outport
  wires:
  In1/1 -> multiplier31/1
  In2/1 -> multiplier31/2
  multiplier31/1 -> Out1/1

== system gm_FCS_MPC_3Phase_SPMSM_TEST1/Microcontroller Software/Subsystem1/MATLAB Function/multiplier32 ==
  In1 : Inport
  In2 : Inport  Port=2
  multiplier32 : Product  Inputs=**  OutDataTypeStr=single  SampleTime=1e-08
  Out1 : Outport
  wires:
  In1/1 -> multiplier32/1
  In2/1 -> multiplier32/2
  multiplier32/1 -> Out1/1

== system gm_FCS_MPC_3Phase_SPMSM_TEST1/Microcontroller Software/Subsystem1/MATLAB Function/multiplier33 ==
  In1 : Inport
  In2 : Inport  Port=2
  multiplier33 : Product  Inputs=**  OutDataTypeStr=single  SampleTime=1e-08
  Out1 : Outport
  wires:
  In1/1 -> multiplier33/1
  In2/1 -> multiplier33/2
  multiplier33/1 -> Out1/1

== system gm_FCS_MPC_3Phase_SPMSM_TEST1/Microcontroller Software/Subsystem1/MATLAB Function/multiplier34 ==
  In1 : Inport
  In2 : Inport  Port=2
  multiplier34 : Product  Inputs=**  OutDataTypeStr=single  SampleTime=1e-08
  Out1 : Outport
  wires:
  In1/1 -> multiplier34/1
  In2/1 -> multiplier34/2
  multiplier34/1 -> Out1/1

== system gm_FCS_MPC_3Phase_SPMSM_TEST1/Microcontroller Software/Subsystem1/MATLAB Function/multiplier35 ==
  In1 : Inport
  In2 : Inport  Port=2
  multiplier35 : Product  Inputs=**  OutDataTypeStr=single  SampleTime=1e-08
  Out1 : Outport
  wires:
  In1/1 -> multiplier35/1
  In2/1 -> multiplier35/2
  multiplier35/1 -> Out1/1

== system gm_FCS_MPC_3Phase_SPMSM_TEST1/Microcontroller Software/Subsystem1/MATLAB Function/multiplier36 ==
  In1 : Inport
  In2 : Inport  Port=2
  multiplier36 : Product  Inputs=**  OutDataTypeStr=single  SampleTime=1e-08
  Out1 : Outport
  wires:
  In1/1 -> multiplier36/1
  In2/1 -> multiplier36/2
  multiplier36/1 -> Out1/1

== system gm_FCS_MPC_3Phase_SPMSM_TEST1/Microcontroller Software/Subsystem1/MATLAB Function/multiplier37 ==
  In1 : Inport
  In2 : Inport  Port=2
  multiplier37 : Product  Inputs=**  OutDataTypeStr=single  SampleTime=1e-08
  Out1 : Outport
  wires:
  In1/1 -> multiplier37/1
  In2/1 -> multiplier37/2
  multiplier37/1 -> Out1/1

== system gm_FCS_MPC_3Phase_SPMSM_TEST1/Microcontroller Software/Subsystem1/MATLAB Function/multiplier38 ==
  In1 : Inport
  In2 : Inport  Port=2
  multiplier38 : Product  Inputs=**  OutDataTypeStr=single  SampleTime=1e-08
  Out1 : Outport
  wires:
  In1/1 -> multiplier38/1
  In2/1 -> multiplier38/2
  multiplier38/1 -> Out1/1

== system gm_FCS_MPC_3Phase_SPMSM_TEST1/Microcontroller Software/Subsystem1/MATLAB Function/multiplier39 ==
  In1 : Inport
  In2 : Inport  Port=2
  multiplier39 : Product  Inputs=**  OutDataTypeStr=single  SampleTime=1e-08
  Out1 : Outport
  wires:
  In1/1 -> multiplier39/1
  In2/1 -> multiplier39/2
  multiplier39/1 -> Out1/1

== system gm_FCS_MPC_3Phase_SPMSM_TEST1/Microcontroller Software/Subsystem1/MATLAB Function/multiplier4 ==
  In1 : Inport
  In2 : Inport  Port=2
  multiplier4 : Product  Inputs=**  OutDataTypeStr=single  SampleTime=1e-08
  Out1 : Outport
  wires:
  In1/1 -> multiplier4/1
  In2/1 -> multiplier4/2
  multiplier4/1 -> Out1/1

== system gm_FCS_MPC_3Phase_SPMSM_TEST1/Microcontroller Software/Subsystem1/MATLAB Function/multiplier40 ==
  In1 : Inport
  In2 : Inport  Port=2
  multiplier40 : Product  Inputs=**  OutDataTypeStr=single  SampleTime=1e-08
  Out1 : Outport
  wires:
  In1/1 -> multiplier40/1
  In2/1 -> multiplier40/2
  multiplier40/1 -> Out1/1

== system gm_FCS_MPC_3Phase_SPMSM_TEST1/Microcontroller Software/Subsystem1/MATLAB Function/multiplier41 ==
  In1 : Inport
  In2 : Inport  Port=2
  multiplier41 : Product  Inputs=**  OutDataTypeStr=single  SampleTime=1e-08
  Out1 : Outport
  wires:
  In1/1 -> multiplier41/1
  In2/1 -> multiplier41/2
  multiplier41/1 -> Out1/1

== system gm_FCS_MPC_3Phase_SPMSM_TEST1/Microcontroller Software/Subsystem1/MATLAB Function/multiplier42 ==
  In1 : Inport
  In2 : Inport  Port=2
  multiplier42 : Product  Inputs=**  OutDataTypeStr=single  SampleTime=1e-08
  Out1 : Outport
  wires:
  In1/1 -> multiplier42/1
  In2/1 -> multiplier42/2
  multiplier42/1 -> Out1/1

== system gm_FCS_MPC_3Phase_SPMSM_TEST1/Microcontroller Software/Subsystem1/MATLAB Function/multiplier43 ==
  In1 : Inport
  In2 : Inport  Port=2
  multiplier43 : Product  Inputs=**  OutDataTypeStr=single  SampleTime=1e-08
  Out1 : Outport
  wires:
  In1/1 -> multiplier43/1
  In2/1 -> multiplier43/2
  multiplier43/1 -> Out1/1

== system gm_FCS_MPC_3Phase_SPMSM_TEST1/Microcontroller Software/Subsystem1/MATLAB Function/multiplier44 ==
  In1 : Inport
  In2 : Inport  Port=2
  multiplier44 : Product  Inputs=**  OutDataTypeStr=single  SampleTime=1e-08
  Out1 : Outport
  wires:
  In1/1 -> multiplier44/1
  In2/1 -> multiplier44/2
  multiplier44/1 -> Out1/1

== system gm_FCS_MPC_3Phase_SPMSM_TEST1/Microcontroller Software/Subsystem1/MATLAB Function/multiplier45 ==
  In1 : Inport
  In2 : Inport  Port=2
  multiplier45 : Product  Inputs=**  OutDataTypeStr=single  SampleTime=1e-08
  Out1 : Outport
  wires:
  In1/1 -> multiplier45/1
  In2/1 -> multiplier45/2
  multiplier45/1 -> Out1/1

== system gm_FCS_MPC_3Phase_SPMSM_TEST1/Microcontroller Software/Subsystem1/MATLAB Function/multiplier46 ==
  In1 : Inport
  In2 : Inport  Port=2
  multiplier46 : Product  Inputs=**  OutDataTypeStr=single  SampleTime=1e-08
  Out1 : Outport
  wires:
  In1/1 -> multiplier46/1
  In2/1 -> multiplier46/2
  multiplier46/1 -> Out1/1

== system gm_FCS_MPC_3Phase_SPMSM_TEST1/Microcontroller Software/Subsystem1/MATLAB Function/multiplier47 ==
  In1 : Inport
  In2 : Inport  Port=2
  multiplier47 : Product  Inputs=**  OutDataTypeStr=single  SampleTime=1e-08
  Out1 : Outport
  wires:
  In1/1 -> multiplier47/1
  In2/1 -> multiplier47/2
  multiplier47/1 -> Out1/1

== system gm_FCS_MPC_3Phase_SPMSM_TEST1/Microcontroller Software/Subsystem1/MATLAB Function/multiplier48 ==
  In1 : Inport
  In2 : Inport  Port=2
  multiplier48 : Product  Inputs=**  OutDataTypeStr=single  SampleTime=1e-08
  Out1 : Outport
  wires:
  In1/1 -> multiplier48/1
  In2/1 -> multiplier48/2
  multiplier48/1 -> Out1/1

== system gm_FCS_MPC_3Phase_SPMSM_TEST1/Microcontroller Software/Subsystem1/MATLAB Function/multiplier49 ==
  In1 : Inport
  In2 : Inport  Port=2
  multiplier49 : Product  Inputs=**  OutDataTypeStr=single  SampleTime=1e-08
  Out1 : Outport
  wires:
  In1/1 -> multiplier49/1
  In2/1 -> multiplier49/2
  multiplier49/1 -> Out1/1

== system gm_FCS_MPC_3Phase_SPMSM_TEST1/Microcontroller Software/Subsystem1/MATLAB Function/multiplier5 ==
  In1 : Inport
  In2 : Inport  Port=2
  multiplier5 : Product  Inputs=**  OutDataTypeStr=single  SampleTime=1e-08
  Out1 : Outport
  wires:
  In1/1 -> multiplier5/1
  In2/1 -> multiplier5/2
  multiplier5/1 -> Out1/1

== system gm_FCS_MPC_3Phase_SPMSM_TEST1/Microcontroller Software/Subsystem1/MATLAB Function/multiplier50 ==
  In1 : Inport
  In2 : Inport  Port=2
  multiplier50 : Product  Inputs=**  OutDataTypeStr=single  SampleTime=1e-08
  Out1 : Outport
  wires:
  In1/1 -> multiplier50/1
  In2/1 -> multiplier50/2
  multiplier50/1 -> Out1/1

== system gm_FCS_MPC_3Phase_SPMSM_TEST1/Microcontroller Software/Subsystem1/MATLAB Function/multiplier51 ==
  In1 : Inport
  In2 : Inport  Port=2
  multiplier51 : Product  Inputs=**  OutDataTypeStr=single  SampleTime=1e-08
  Out1 : Outport
  wires:
  In1/1 -> multiplier51/1
  In2/1 -> multiplier51/2
  multiplier51/1 -> Out1/1

== system gm_FCS_MPC_3Phase_SPMSM_TEST1/Microcontroller Software/Subsystem1/MATLAB Function/multiplier52 ==
  In1 : Inport
  In2 : Inport  Port=2
  multiplier52 : Product  Inputs=**  OutDataTypeStr=single  SampleTime=1e-08
  Out1 : Outport
  wires:
  In1/1 -> multiplier52/1
  In2/1 -> multiplier52/2
  multiplier52/1 -> Out1/1

== system gm_FCS_MPC_3Phase_SPMSM_TEST1/Microcontroller Software/Subsystem1/MATLAB Function/multiplier53 ==
  In1 : Inport
  In2 : Inport  Port=2
  multiplier53 : Product  Inputs=**  OutDataTypeStr=single  SampleTime=1e-08
  Out1 : Outport
  wires:
  In1/1 -> multiplier53/1
  In2/1 -> multiplier53/2
  multiplier53/1 -> Out1/1

== system gm_FCS_MPC_3Phase_SPMSM_TEST1/Microcontroller Software/Subsystem1/MATLAB Function/multiplier54 ==
  In1 : Inport
  In2 : Inport  Port=2
  multiplier54 : Product  Inputs=**  OutDataTypeStr=single  SampleTime=1e-08
  Out1 : Outport
  wires:
  In1/1 -> multiplier54/1
  In2/1 -> multiplier54/2
  multiplier54/1 -> Out1/1

== system gm_FCS_MPC_3Phase_SPMSM_TEST1/Microcontroller Software/Subsystem1/MATLAB Function/multiplier55 ==
  In1 : Inport
  In2 : Inport  Port=2
  multiplier55 : Product  Inputs=**  OutDataTypeStr=single  SampleTime=1e-08
  Out1 : Outport
  wires:
  In1/1 -> multiplier55/1
  In2/1 -> multiplier55/2
  multiplier55/1 -> Out1/1

== system gm_FCS_MPC_3Phase_SPMSM_TEST1/Microcontroller Software/Subsystem1/MATLAB Function/multiplier56 ==
  In1 : Inport
  In2 : Inport  Port=2
  multiplier56 : Product  Inputs=**  OutDataTypeStr=single  SampleTime=1e-08
  Out1 : Outport
  wires:
  In1/1 -> multiplier56/1
  In2/1 -> multiplier56/2
  multiplier56/1 -> Out1/1

== system gm_FCS_MPC_3Phase_SPMSM_TEST1/Microcontroller Software/Subsystem1/MATLAB Function/multiplier57 ==
  In1 : Inport
  In2 : Inport  Port=2
  multiplier57 : Product  Inputs=**  OutDataTypeStr=single  SampleTime=1e-08
  Out1 : Outport
  wires:
  In1/1 -> multiplier57/1
  In2/1 -> multiplier57/2
  multiplier57/1 -> Out1/1

== system gm_FCS_MPC_3Phase_SPMSM_TEST1/Microcontroller Software/Subsystem1/MATLAB Function/multiplier58 ==
  In1 : Inport
  In2 : Inport  Port=2
  multiplier58 : Product  Inputs=**  OutDataTypeStr=single  SampleTime=1e-08
  Out1 : Outport
  wires:
  In1/1 -> multiplier58/1
  In2/1 -> multiplier58/2
  multiplier58/1 -> Out1/1

== system gm_FCS_MPC_3Phase_SPMSM_TEST1/Microcontroller Software/Subsystem1/MATLAB Function/multiplier59 ==
  In1 : Inport
  In2 : Inport  Port=2
  multiplier59 : Product  Inputs=**  OutDataTypeStr=single  SampleTime=1e-08
  Out1 : Outport
  wires:
  In1/1 -> multiplier59/1
  In2/1 -> multiplier59/2
  multiplier59/1 -> Out1/1

== system gm_FCS_MPC_3Phase_SPMSM_TEST1/Microcontroller Software/Subsystem1/MATLAB Function/multiplier6 ==
  In1 : Inport
  In2 : Inport  Port=2
  multiplier6 : Product  Inputs=**  OutDataTypeStr=single  SampleTime=1e-08
  Out1 : Outport
  wires:
  In1/1 -> multiplier6/1
  In2/1 -> multiplier6/2
  multiplier6/1 -> Out1/1

== system gm_FCS_MPC_3Phase_SPMSM_TEST1/Microcontroller Software/Subsystem1/MATLAB Function/multiplier60 ==
  In1 : Inport
  In2 : Inport  Port=2
  multiplier60 : Product  Inputs=**  OutDataTypeStr=single  SampleTime=1e-08
  Out1 : Outport
  wires:
  In1/1 -> multiplier60/1
  In2/1 -> multiplier60/2
  multiplier60/1 -> Out1/1

== system gm_FCS_MPC_3Phase_SPMSM_TEST1/Microcontroller Software/Subsystem1/MATLAB Function/multiplier61 ==
  In1 : Inport
  In2 : Inport  Port=2
  multiplier61 : Product  Inputs=**  OutDataTypeStr=single  SampleTime=1e-08
  Out1 : Outport
  wires:
  In1/1 -> multiplier61/1
  In2/1 -> multiplier61/2
  multiplier61/1 -> Out1/1

== system gm_FCS_MPC_3Phase_SPMSM_TEST1/Microcontroller Software/Subsystem1/MATLAB Function/multiplier62 ==
  In1 : Inport
  In2 : Inport  Port=2
  multiplier62 : Product  Inputs=**  OutDataTypeStr=single  SampleTime=1e-08
  Out1 : Outport
  wires:
  In1/1 -> multiplier62/1
  In2/1 -> multiplier62/2
  multiplier62/1 -> Out1/1

== system gm_FCS_MPC_3Phase_SPMSM_TEST1/Microcontroller Software/Subsystem1/MATLAB Function/multiplier63 ==
  In1 : Inport
  In2 : Inport  Port=2
  multiplier63 : Product  Inputs=**  OutDataTypeStr=single  SampleTime=1e-08
  Out1 : Outport
  wires:
  In1/1 -> multiplier63/1
  In2/1 -> multiplier63/2
  multiplier63/1 -> Out1/1

== system gm_FCS_MPC_3Phase_SPMSM_TEST1/Microcontroller Software/Subsystem1/MATLAB Function/multiplier64 ==
  In1 : Inport
  In2 : Inport  Port=2
  multiplier64 : Product  Inputs=**  OutDataTypeStr=single  SampleTime=1e-08
  Out1 : Outport
  wires:
  In1/1 -> multiplier64/1
  In2/1 -> multiplier64/2
  multiplier64/1 -> Out1/1

== system gm_FCS_MPC_3Phase_SPMSM_TEST1/Microcontroller Software/Subsystem1/MATLAB Function/multiplier65 ==
  In1 : Inport
  In2 : Inport  Port=2
  multiplier65 : Product  Inputs=**  OutDataTypeStr=single  SampleTime=1e-08
  Out1 : Outport
  wires:
  In1/1 -> multiplier65/1
  In2/1 -> multiplier65/2
  multiplier65/1 -> Out1/1

== system gm_FCS_MPC_3Phase_SPMSM_TEST1/Microcontroller Software/Subsystem1/MATLAB Function/multiplier66 ==
  In1 : Inport
  In2 : Inport  Port=2
  multiplier66 : Product  Inputs=**  OutDataTypeStr=single  SampleTime=1e-08
  Out1 : Outport
  wires:
  In1/1 -> multiplier66/1
  In2/1 -> multiplier66/2
  multiplier66/1 -> Out1/1

== system gm_FCS_MPC_3Phase_SPMSM_TEST1/Microcontroller Software/Subsystem1/MATLAB Function/multiplier67 ==
  In1 : Inport
  In2 : Inport  Port=2
  multiplier67 : Product  Inputs=**  OutDataTypeStr=single  SampleTime=1e-08
  Out1 : Outport
  wires:
  In1/1 -> multiplier67/1
  In2/1 -> multiplier67/2
  multiplier67/1 -> Out1/1

== system gm_FCS_MPC_3Phase_SPMSM_TEST1/Microcontroller Software/Subsystem1/MATLAB Function/multiplier68 ==
  In1 : Inport
  In2 : Inport  Port=2
  multiplier68 : Product  Inputs=**  OutDataTypeStr=single  SampleTime=1e-08
  Out1 : Outport
  wires:
  In1/1 -> multiplier68/1
  In2/1 -> multiplier68/2
  multiplier68/1 -> Out1/1

== system gm_FCS_MPC_3Phase_SPMSM_TEST1/Microcontroller Software/Subsystem1/MATLAB Function/multiplier69 ==
  In1 : Inport
  In2 : Inport  Port=2
  multiplier69 : Product  Inputs=**  OutDataTypeStr=single  SampleTime=1e-08
  Out1 : Outport
  wires:
  In1/1 -> multiplier69/1
  In2/1 -> multiplier69/2
  multiplier69/1 -> Out1/1

== system gm_FCS_MPC_3Phase_SPMSM_TEST1/Microcontroller Software/Subsystem1/MATLAB Function/multiplier7 ==
  In1 : Inport
  In2 : Inport  Port=2
  multiplier7 : Product  Inputs=**  OutDataTypeStr=single  SampleTime=1e-08
  Out1 : Outport
  wires:
  In1/1 -> multiplier7/1
  In2/1 -> multiplier7/2
  multiplier7/1 -> Out1/1

== system gm_FCS_MPC_3Phase_SPMSM_TEST1/Microcontroller Software/Subsystem1/MATLAB Function/multiplier70 ==
  In1 : Inport
  In2 : Inport  Port=2
  multiplier70 : Product  Inputs=**  OutDataTypeStr=single  SampleTime=1e-08
  Out1 : Outport
  wires:
  In1/1 -> multiplier70/1
  In2/1 -> multiplier70/2
  multiplier70/1 -> Out1/1

== system gm_FCS_MPC_3Phase_SPMSM_TEST1/Microcontroller Software/Subsystem1/MATLAB Function/multiplier71 ==
  In1 : Inport
  In2 : Inport  Port=2
  multiplier71 : Product  Inputs=**  OutDataTypeStr=single  SampleTime=1e-08
  Out1 : Outport
  wires:
  In1/1 -> multiplier71/1
  In2/1 -> multiplier71/2
  multiplier71/1 -> Out1/1

== system gm_FCS_MPC_3Phase_SPMSM_TEST1/Microcontroller Software/Subsystem1/MATLAB Function/multiplier72 ==
  In1 : Inport
  In2 : Inport  Port=2
  multiplier72 : Product  Inputs=**  OutDataTypeStr=single  SampleTime=1e-08
  Out1 : Outport
  wires:
  In1/1 -> multiplier72/1
  In2/1 -> multiplier72/2
  multiplier72/1 -> Out1/1

== system gm_FCS_MPC_3Phase_SPMSM_TEST1/Microcontroller Software/Subsystem1/MATLAB Function/multiplier73 ==
  In1 : Inport
  In2 : Inport  Port=2
  multiplier73 : Product  Inputs=**  OutDataTypeStr=single  SampleTime=1e-08
  Out1 : Outport
  wires:
  In1/1 -> multiplier73/1
  In2/1 -> multiplier73/2
  multiplier73/1 -> Out1/1

== system gm_FCS_MPC_3Phase_SPMSM_TEST1/Microcontroller Software/Subsystem1/MATLAB Function/multiplier74 ==
  In1 : Inport
  In2 : Inport  Port=2
  multiplier74 : Product  Inputs=**  OutDataTypeStr=single  SampleTime=1e-08
  Out1 : Outport
  wires:
  In1/1 -> multiplier74/1
  In2/1 -> multiplier74/2
  multiplier74/1 -> Out1/1

== system gm_FCS_MPC_3Phase_SPMSM_TEST1/Microcontroller Software/Subsystem1/MATLAB Function/multiplier75 ==
  In1 : Inport
  In2 : Inport  Port=2
  multiplier75 : Product  Inputs=**  OutDataTypeStr=single  SampleTime=1e-08
  Out1 : Outport
  wires:
  In1/1 -> multiplier75/1
  In2/1 -> multiplier75/2
  multiplier75/1 -> Out1/1

== system gm_FCS_MPC_3Phase_SPMSM_TEST1/Microcontroller Software/Subsystem1/MATLAB Function/multiplier76 ==
  In1 : Inport
  In2 : Inport  Port=2
  multiplier76 : Product  Inputs=**  OutDataTypeStr=single  SampleTime=1e-08
  Out1 : Outport
  wires:
  In1/1 -> multiplier76/1
  In2/1 -> multiplier76/2
  multiplier76/1 -> Out1/1

== system gm_FCS_MPC_3Phase_SPMSM_TEST1/Microcontroller Software/Subsystem1/MATLAB Function/multiplier77 ==
  In1 : Inport
  In2 : Inport  Port=2
  multiplier77 : Product  Inputs=**  OutDataTypeStr=single  SampleTime=1e-08
  Out1 : Outport
  wires:
  In1/1 -> multiplier77/1
  In2/1 -> multiplier77/2
  multiplier77/1 -> Out1/1

== system gm_FCS_MPC_3Phase_SPMSM_TEST1/Microcontroller Software/Subsystem1/MATLAB Function/multiplier78 ==
  In1 : Inport
  In2 : Inport  Port=2
  multiplier78 : Product  Inputs=**  OutDataTypeStr=single  SampleTime=1e-08
  Out1 : Outport
  wires:
  In1/1 -> multiplier78/1
  In2/1 -> multiplier78/2
  multiplier78/1 -> Out1/1

== system gm_FCS_MPC_3Phase_SPMSM_TEST1/Microcontroller Software/Subsystem1/MATLAB Function/multiplier79 ==
  In1 : Inport
  In2 : Inport  Port=2
  multiplier79 : Product  Inputs=**  OutDataTypeStr=single  SampleTime=1e-08
  Out1 : Outport
  wires:
  In1/1 -> multiplier79/1
  In2/1 -> multiplier79/2
  multiplier79/1 -> Out1/1

== system gm_FCS_MPC_3Phase_SPMSM_TEST1/Microcontroller Software/Subsystem1/MATLAB Function/multiplier8 ==
  In1 : Inport
  In2 : Inport  Port=2
  multiplier8 : Product  Inputs=**  OutDataTypeStr=single  SampleTime=1e-08
  Out1 : Outport
  wires:
  In1/1 -> multiplier8/1
  In2/1 -> multiplier8/2
  multiplier8/1 -> Out1/1

== system gm_FCS_MPC_3Phase_SPMSM_TEST1/Microcontroller Software/Subsystem1/MATLAB Function/multiplier80 ==
  In1 : Inport
  In2 : Inport  Port=2
  multiplier80 : Product  Inputs=**  OutDataTypeStr=single  SampleTime=1e-08
  Out1 : Outport
  wires:
  In1/1 -> multiplier80/1
  In2/1 -> multiplier80/2
  multiplier80/1 -> Out1/1

== system gm_FCS_MPC_3Phase_SPMSM_TEST1/Microcontroller Software/Subsystem1/MATLAB Function/multiplier81 ==
  In1 : Inport
  In2 : Inport  Port=2
  multiplier81 : Product  Inputs=**  OutDataTypeStr=single  SampleTime=1e-08
  Out1 : Outport
  wires:
  In1/1 -> multiplier81/1
  In2/1 -> multiplier81/2
  multiplier81/1 -> Out1/1

== system gm_FCS_MPC_3Phase_SPMSM_TEST1/Microcontroller Software/Subsystem1/MATLAB Function/multiplier82 ==
  In1 : Inport
  In2 : Inport  Port=2
  multiplier82 : Product  Inputs=**  OutDataTypeStr=single  SampleTime=1e-08
  Out1 : Outport
  wires:
  In1/1 -> multiplier82/1
  In2/1 -> multiplier82/2
  multiplier82/1 -> Out1/1

== system gm_FCS_MPC_3Phase_SPMSM_TEST1/Microcontroller Software/Subsystem1/MATLAB Function/multiplier83 ==
  In1 : Inport
  In2 : Inport  Port=2
  multiplier83 : Product  Inputs=**  OutDataTypeStr=single  SampleTime=1e-08
  Out1 : Outport
  wires:
  In1/1 -> multiplier83/1
  In2/1 -> multiplier83/2
  multiplier83/1 -> Out1/1

== system gm_FCS_MPC_3Phase_SPMSM_TEST1/Microcontroller Software/Subsystem1/MATLAB Function/multiplier84 ==
  In1 : Inport
  In2 : Inport  Port=2
  multiplier84 : Product  Inputs=**  OutDataTypeStr=single  SampleTime=1e-08
  Out1 : Outport
  wires:
  In1/1 -> multiplier84/1
  In2/1 -> multiplier84/2
  multiplier84/1 -> Out1/1

== system gm_FCS_MPC_3Phase_SPMSM_TEST1/Microcontroller Software/Subsystem1/MATLAB Function/multiplier85 ==
  In1 : Inport
  In2 : Inport  Port=2
  multiplier85 : Product  Inputs=**  OutDataTypeStr=single  SampleTime=1e-08
  Out1 : Outport
  wires:
  In1/1 -> multiplier85/1
  In2/1 -> multiplier85/2
  multiplier85/1 -> Out1/1

== system gm_FCS_MPC_3Phase_SPMSM_TEST1/Microcontroller Software/Subsystem1/MATLAB Function/multiplier86 ==
  In1 : Inport
  In2 : Inport  Port=2
  multiplier86 : Product  Inputs=**  OutDataTypeStr=single  SampleTime=1e-08
  Out1 : Outport
  wires:
  In1/1 -> multiplier86/1
  In2/1 -> multiplier86/2
  multiplier86/1 -> Out1/1

== system gm_FCS_MPC_3Phase_SPMSM_TEST1/Microcontroller Software/Subsystem1/MATLAB Function/multiplier87 ==
  In1 : Inport
  In2 : Inport  Port=2
  multiplier87 : Product  Inputs=**  OutDataTypeStr=single  SampleTime=1e-08
  Out1 : Outport
  wires:
  In1/1 -> multiplier87/1
  In2/1 -> multiplier87/2
  multiplier87/1 -> Out1/1

== system gm_FCS_MPC_3Phase_SPMSM_TEST1/Microcontroller Software/Subsystem1/MATLAB Function/multiplier88 ==
  In1 : Inport
  In2 : Inport  Port=2
  multiplier88 : Product  Inputs=**  OutDataTypeStr=single  SampleTime=1e-08
  Out1 : Outport
  wires:
  In1/1 -> multiplier88/1
  In2/1 -> multiplier88/2
  multiplier88/1 -> Out1/1

== system gm_FCS_MPC_3Phase_SPMSM_TEST1/Microcontroller Software/Subsystem1/MATLAB Function/multiplier89 ==
  In1 : Inport
  In2 : Inport  Port=2
  multiplier89 : Product  Inputs=**  OutDataTypeStr=single  SampleTime=1e-08
  Out1 : Outport
  wires:
  In1/1 -> multiplier89/1
  In2/1 -> multiplier89/2
  multiplier89/1 -> Out1/1

== system gm_FCS_MPC_3Phase_SPMSM_TEST1/Microcontroller Software/Subsystem1/MATLAB Function/multiplier9 ==
  In1 : Inport
  In2 : Inport  Port=2
  multiplier9 : Product  Inputs=**  OutDataTypeStr=single  SampleTime=1e-08
  Out1 : Outport
  wires:
  In1/1 -> multiplier9/1
  In2/1 -> multiplier9/2
  multiplier9/1 -> Out1/1

== system gm_FCS_MPC_3Phase_SPMSM_TEST1/Microcontroller Software/Subsystem1/MATLAB Function/square ==
  In1 : Inport
  In2 : Inport  Port=2
  square : Product  Inputs=**  OutDataTypeStr=single  SampleTime=1e-08
  Out1 : Outport
  wires:
  In1/1 -> square/1
  In2/1 -> square/2
  square/1 -> Out1/1

== system gm_FCS_MPC_3Phase_SPMSM_TEST1/Microcontroller Software/Subsystem1/MATLAB Function/square1 ==
  In1 : Inport
  In2 : Inport  Port=2
  square1 : Product  Inputs=**  OutDataTypeStr=single  SampleTime=1e-08
  Out1 : Outport
  wires:
  In1/1 -> square1/1
  In2/1 -> square1/2
  square1/1 -> Out1/1

== system gm_FCS_MPC_3Phase_SPMSM_TEST1/Microcontroller Software/Subsystem1/MATLAB Function/square10 ==
  In1 : Inport
  In2 : Inport  Port=2
  square10 : Product  Inputs=**  OutDataTypeStr=single  SampleTime=1e-08
  Out1 : Outport
  wires:
  In1/1 -> square10/1
  In2/1 -> square10/2
  square10/1 -> Out1/1
